simulink model "fifteen_level"  (Simulink 7.5)
settings: Solver=ode23tb  StartTime=0.0  StopTime=0.1  MaxStep=5e-6  RelTol=1e-3
libraries: powerlib x25
settings Model: Creator=GURU  LastModifiedBy=lenova
settings DebuggingCC: StrictBusMsg=Warning

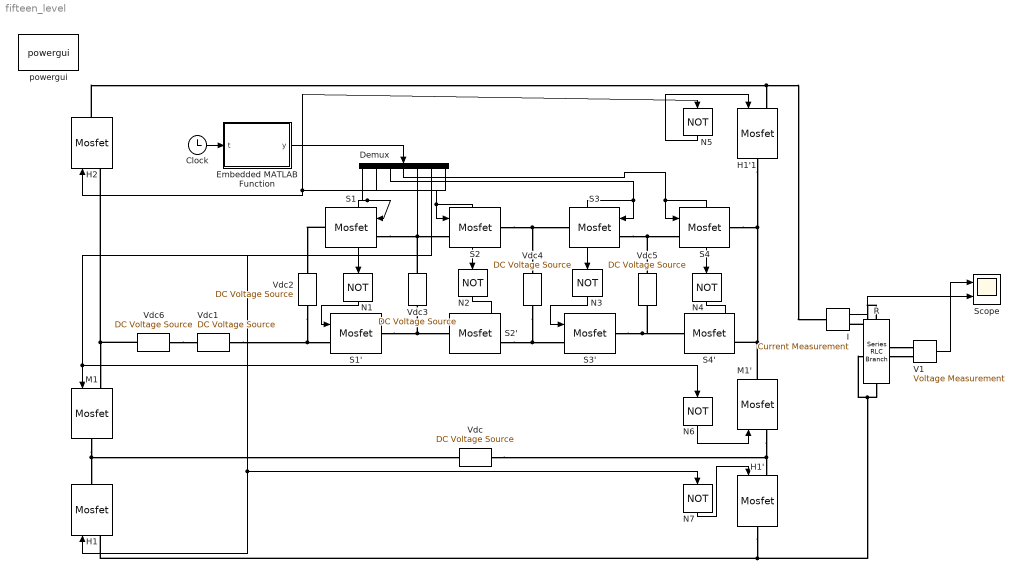
== system fifteen_level ==
  Clock : Clock
      settings: Decimation=10
  Demux : Demux  Outputs=7
  Embedded MATLAB Function : Stateflow chart  TreatAsAtomicUnit=on
  H1 : powerlib/Power Electronics/Mosfet  DialogController=POWERSYS.PowerSysDialog  SystemSampleTime=-1  Ron=0.1  Lon=0  Rd=0.01  Vfd=0  IC=0  Rs=1e5  Cs=inf  Measurements=off
  H1' : powerlib/Power Electronics/Mosfet  DialogController=POWERSYS.PowerSysDialog  SystemSampleTime=-1  Ron=0.1  Lon=0  Rd=0.01  Vfd=0  IC=0  Rs=1e5  Cs=inf  Measurements=off
  H1'1 : powerlib/Power Electronics/Mosfet  DialogController=POWERSYS.PowerSysDialog  SystemSampleTime=-1  Ron=0.1  Lon=0  Rd=0.01  Vfd=0  IC=0  Rs=1e5  Cs=inf  Measurements=off
  H2 : powerlib/Power Electronics/Mosfet  DialogController=POWERSYS.PowerSysDialog  SystemSampleTime=-1  Ron=0.1  Lon=0  Rd=0.01  Vfd=0  IC=0  Rs=1e5  Cs=inf  Measurements=off
  I : powerlib/Measurements/Current Measurement  DialogController=POWERSYS.PowerSysDialog  SystemSampleTime=-1  PhasorSimulation=off  OutputType=Complex  PSBequivalent=0
  M1 : powerlib/Power Electronics/Mosfet  DialogController=POWERSYS.PowerSysDialog  SystemSampleTime=-1  Ron=0.1  Lon=0  Rd=0.01  Vfd=0  IC=0  Rs=1e5  Cs=inf  Measurements=off
  M1' : powerlib/Power Electronics/Mosfet  DialogController=POWERSYS.PowerSysDialog  SystemSampleTime=-1  Ron=0.1  Lon=0  Rd=0.01  Vfd=0  IC=0  Rs=1e5  Cs=inf  Measurements=off
  N{1..7} (7 alike) : Logic  Operator=NOT  AllPortsSameDT=off  OutDataTypeMode=boolean  LogicDataType=fixdt(0, 8)  OutDataTypeStr=boolean
  R : powerlib/Elements/Series RLC Branch  DialogController=POWERSYS.PowerSysDialog  PhysicalDomain=powersysdomain  SubClassName=unknown  LeftPortType=p1  RightPortType=p1  LConnTagsString=__new0  RConnTagsString=__new0  BranchType=RL  Resistance=10  Inductance=1e-3  SetiL0=off  InitialCurrent=0  Capacitance=1e-6  Setx0=off  InitialVoltage=0  Measurements=None
  S{1..4} (4 alike) : powerlib/Power Electronics/Mosfet  DialogController=POWERSYS.PowerSysDialog  SystemSampleTime=-1  Ron=0.1  Lon=0  Rd=0.01  Vfd=0  IC=0  Rs=1e5  Cs=inf  Measurements=off
  S1' : powerlib/Power Electronics/Mosfet  DialogController=POWERSYS.PowerSysDialog  SystemSampleTime=-1  Ron=0.1  Lon=0  Rd=0.01  Vfd=0  IC=0  Rs=1e5  Cs=inf  Measurements=off
  S2' : powerlib/Power Electronics/Mosfet  DialogController=POWERSYS.PowerSysDialog  SystemSampleTime=-1  Ron=0.1  Lon=0  Rd=0.01  Vfd=0  IC=0  Rs=1e5  Cs=inf  Measurements=off
  S3' : powerlib/Power Electronics/Mosfet  DialogController=POWERSYS.PowerSysDialog  SystemSampleTime=-1  Ron=0.1  Lon=0  Rd=0.01  Vfd=0  IC=0  Rs=1e5  Cs=inf  Measurements=off
  S4' : powerlib/Power Electronics/Mosfet  DialogController=POWERSYS.PowerSysDialog  SystemSampleTime=-1  Ron=0.1  Lon=0  Rd=0.01  Vfd=0  IC=0  Rs=1e5  Cs=inf  Measurements=off
  Scope : Scope  NumInputPorts=2
      settings: YMin=-350~-35  YMax=350~35  MaxDataPoints=5000000
  V1 : powerlib/Measurements/Voltage Measurement  DialogController=POWERSYS.PowerSysDialog  SystemSampleTime=-1  PhasorSimulation=off  OutputType=Complex  PSBequivalent=0
  Vdc{,1..6} (7 alike) : powerlib/Electrical Sources/DC Voltage Source  DialogController=POWERSYS.PowerSysDialog  SystemSampleTime=-1  Amplitude=(230*sqrt(2)/7)  Measurements=None
  powergui : powerlib/powergui  Priority=1  SystemSampleTime=-1  SimulationMode=Continuous  SampleTime=50e-6  frequency=60  SPID=off  DisableSnubberDevices=off  DisableRonSwitches=off  DisableVfSwitches=off  SwTol=0  Interpol=off  frequencyindice=0  echomessages=off  HookPort=off  DisplayEquations=off  FunctionMessages=off  EnableUseOfTLC=off  x0status=blocks  RestoreLinks=warning  ResistiveCurrentMeasurement=off  Frange=[0:2:500]  Ylog=off  Xlog=on  ShowGrid=off  save=off  variable=ZData  structure=ScopeData  ZoomFFT=off  StartTime=0.0  cycles=5  DisplayStyle=1  fundamental=50  FreqAxis=off  MaxFrequency=1000  frequencyindicesteady=1  RmsSteady=1  display=off  Ts=0  methode=off
  wires:
  V1/1 -> Scope/1
  I/1 -> Scope/2
  Clock/1 -> Embedded MATLAB Function/1(t)
  N1/1 -> S1'/1
  N2/1 -> S2'/1
  N3/1 -> S3'/1
  N4/1 -> S4'/1
  N6/1 -> M1'/1
  N7/1 -> H1'/1
  N5/1 -> H1'1/1
  Embedded MATLAB Function/1(y) -> Demux/1
  Demux/1 -> S1/1, N1/1
  Demux/2 -> S2/1, N2/1
  Demux/3 -> S3/1, N3/1
  Demux/4 -> S4/1, N4/1
  Demux/5 -> H1/1, N7/1
  Demux/6 -> M1/1, N6/1
  Demux/7 -> H2/1, N5/1
  connections:
  R/LConn1 -- I/RConn1 -- V1/LConn1
  S1/RConn1 -- Vdc2/LConn1
  Vdc1/LConn1 -- S1'/LConn1 -- Vdc2/RConn1
  Vdc6/LConn1 -- Vdc1/RConn1
  S1/LConn1 -- S2/LConn1 -- Vdc3/RConn1
  S1'/RConn1 -- S2'/RConn1 -- Vdc3/LConn1
  S2/RConn1 -- S3/RConn1 -- Vdc4/LConn1
  S2'/LConn1 -- S3'/LConn1 -- Vdc4/RConn1
  S3/LConn1 -- S4/LConn1 -- Vdc5/RConn1
  S3'/RConn1 -- S4'/RConn1 -- Vdc5/LConn1
  S4/RConn1 -- S4'/LConn1 -- M1'/RConn1 -- H1'1/RConn1
  M1'/LConn1 -- H1'/LConn1 -- Vdc/RConn1
  Vdc6/RConn1 -- M1/LConn1 -- H2/LConn1
  M1/RConn1 -- H1/RConn1 -- Vdc/LConn1
  H2/RConn1 -- H1'1/LConn1 -- I/LConn1
  R/RConn1 -- V1/LConn2 -- H1/LConn1 -- H1'/RConn1

== matlab function Embedded MATLAB Function ==
  data: t input double; y output double
function y = fcn(t)
%#eml
f=50;
r=sin(2*pi*f*t);
ar=abs(r);

if ar<0.5/7
    s1=0;s2=0;s3=0;s4=0;
       elseif ar<1.5/7 
           s1=0;s2=0;s3=0;s4=0;
            elseif ar<2.5/7 
                s1=0;s2=0;s3=0;s4=1;
                 elseif ar<3.5/7 
                     s1=0;s2=0;s3=0;s4=0;
                      elseif ar<4.5/7 
                          s1=1;s2=0;s3=0;s4=1;
                           elseif ar<5.5/7 
                               s1=1;s2=0;s3=0;s4=0;
                                elseif ar<6.5/7 
                                    s1=1;s2=0;s3=1;s4=1;
else
            s1=1;s2=0;s3=1;s4=0;
       
 end
    if r>0
        
            if ar<0.5/7
                 h1=0;m1=0;h2=0;
            elseif ar<1.5/7
                h1=1;m1=0;h2=0;         
            else
                h1=1;m1=0;h2=1;
            end
    else
        
        if ar<0.5/7
                h1=1;m1=1;h2=1;
        elseif ar<1.5/7
                 h1=0;m1=1;h2=1;
            else
                h1=0;m1=1;h2=0;
            end
        end
y = [s1 s2 s3 s4 h1 m1 h2];
